simulink model "P2_Q5"  (R2023a)
settings: Solver=VariableStepAuto  StartTime=0.0  StopTime=50  RelTol=1e-3
settings Model: Creator=asus  LastModifiedBy=asus

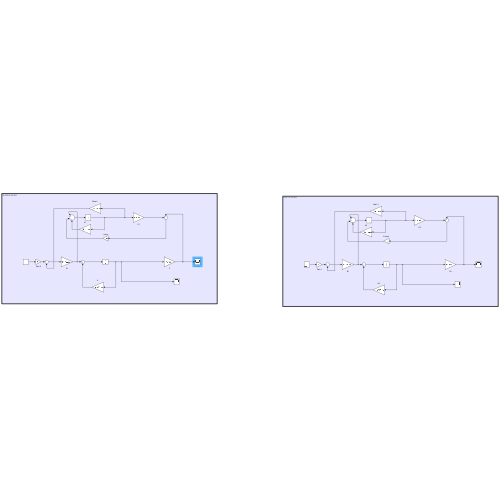
[thumbnail: Simulink's stored preview of the top-level diagram]
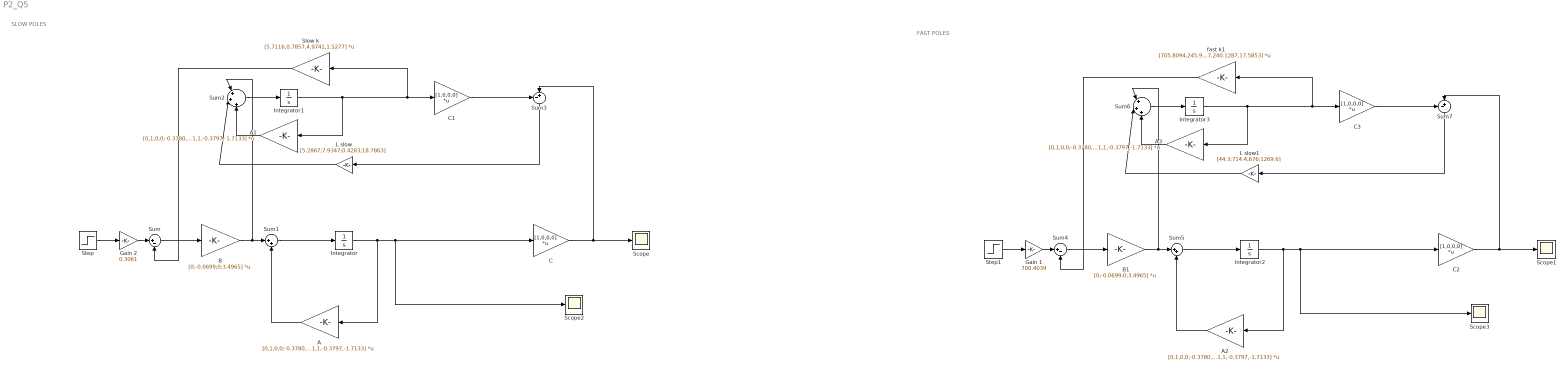
== system P2_Q5 ==
  note: SLOW POLES
  note: FAST POLES
  A{,1..3} (4 alike) : Gain  Gain=[0,1,0,0;-0.3780,0,7.0147,0.0343;0,0,0,1;18.9001,1,-0.3797,-1.7133]  Multiplication=Matrix(K*u) (u vector)
  B : Gain  Gain=[0;-0.0699;0;3.4965]  Multiplication=Matrix(K*u) (u vector)
  B1 : Gain  Gain=[0;-0.0699;0;3.4965]  Multiplication=Matrix(K*u) (u vector)
  C{,1..3} (4 alike) : Gain  Gain=[1,0,0,0]  Multiplication=Matrix(K*u) (u vector)
  Gain 1 : Gain  Gain=700.4039
  Gain 2 : Gain  Gain=0.3061
  Integrator{,1..3} (4 alike) : Integrator
  L slow : Gain  Gain=[5.2867;7.9347;0.4283;18.7863]
  L slow1 : Gain  Gain=[44.3;714.4;676;1269.6]
  Scope{,1..3} (4 alike) : Scope
  Slow k : Gain  Gain=[5.7116,0.7857,4.9741,1.5277]  Multiplication=Matrix(K*u) (u vector)
  Step : Step  Time=0  After=0.1  SampleTime=0
  Step1 : Step  Time=0  After=0.1  SampleTime=0
  Sum : Sum  Inputs=|+-
  Sum1 : Sum  Inputs=|++
  Sum2 : Sum  Inputs=|+|+|+
  Sum3 : Sum  Inputs=-+|
  Sum4 : Sum  Inputs=|+-
  Sum5 : Sum  Inputs=|++
  Sum6 : Sum  Inputs=|+|+|+
  Sum7 : Sum  Inputs=-+|
  fast k1 : Gain  Gain=[705.8094,245.9577,240.1287,17.5853]  Multiplication=Matrix(K*u) (u vector)
  wires:
  Sum1/1 -> Integrator/1
  Sum3/1 -> L slow/1
  A1/1 -> Sum2/3
  L slow/1 -> Sum2/2
  Integrator1/1 -> A1/1, Slow k/1, C1/1
  Slow k/1 -> Sum/2
  Step/1 -> Gain 2/1
  Gain 2/1 -> Sum/1
  C/1 -> Scope/1, Sum3/2
  C1/1 -> Sum3/1
  Sum/1 -> B/1
  B/1 -> Sum1/1, Sum2/1
  Sum2/1 -> Integrator1/1
  Integrator/1 -> A/1, C/1, Scope2/1
  A/1 -> Sum1/2
  Sum4/1 -> B1/1
  Step1/1 -> Gain 1/1
  A2/1 -> Sum5/2
  L slow1/1 -> Sum6/2
  Integrator2/1 -> A2/1, C2/1, Scope3/1
  Sum5/1 -> Integrator2/1
  B1/1 -> Sum5/1, Sum6/1
  fast k1/1 -> Sum4/2
  Gain 1/1 -> Sum4/1
  C3/1 -> Sum7/1
  A3/1 -> Sum6/3
  C2/1 -> Scope1/1, Sum7/2
  Sum7/1 -> L slow1/1
  Integrator3/1 -> A3/1, fast k1/1, C3/1
  Sum6/1 -> Integrator3/1
